simulink model "Problem3_Week2"  (R2020b)
settings: Solver=VariableStepAuto  StartTime=0.0  StopTime=10.0  RelTol=1e-3
model workspace (MAT data in the model file):
  Ki = Simulink.Parameter
  Ki.Value = 40
  Ki.DataType = 'auto'
  Ki.Dimensions = [1 1]
  Kp = Simulink.Parameter
  Kp.Value = 5000
  Kp.DataType = 'auto'
  Kp.Dimensions = [1 1]
  b = Simulink.Parameter
  b.Value = 50
  b.DataType = 'auto'
  b.Dimensions = [1 1]
  m = Simulink.Parameter
  m.Value = 1000
  m.DataType = 'auto'
  m.Dimensions = [1 1]
  u = Simulink.Parameter
  u.Value = 500
  u.DataType = 'auto'
  u.Dimensions = [1 1]
settings Model: DataDictionary=Data_Dictionary.sldd  Creator=hp  LastModifiedBy=hp
settings DebuggingCC: ModelReferenceExtraNoncontSigs=none

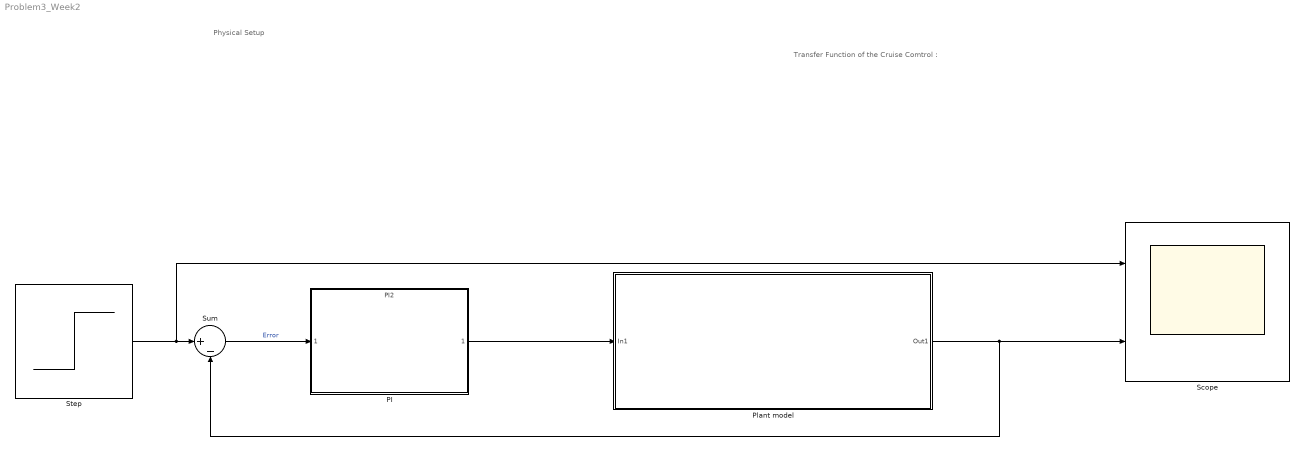
== system Problem3_Week2 ==
  note: Physical Setup
  note: Transfer Function of the Cruise Comtrol :
  PI : ModelReference  ModelNameDialog=PI2  SimulationMode=Normal  ModelReferenceVersion=1.6
  Plant model : Subsystem
  Scope : Scope  NumInputPorts=2
  Step : Step  Time=0  After=u  SampleTime=0
  Sum : Sum  Inputs=|+-
  wires:
  Plant model/1(Out1) -> Sum/2, Scope/2
  Step/1 -> Sum/1, Scope/1
  PI/1 -> Plant model/1(In1)
  Sum/1 -> PI/1  "Error"

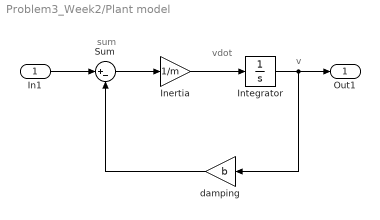
== system Problem3_Week2/Plant model ==
  note: vdot
  note: sum
  note: v
  In1 : Inport
  Inertia : Gain  Gain=1/m
  Integrator : Integrator
  Sum : Sum  Inputs=|+-
  damping : Gain  Gain=b
  Out1 : Outport
  wires:
  In1/1 -> Sum/1
  Sum/1 -> Inertia/1
  Inertia/1 -> Integrator/1
  damping/1 -> Sum/2
  Integrator/1 -> Out1/1, damping/1
